simulink model "SecRwRtStArmScrnIsPosChk"  (R2018b)
settings: Solver=FixedStepDiscrete  StartTime=0.0  StopTime=10.0  FixedStep=0.01  RelTol=1e-3
undefined symbols (not defined in the file or in its folder): KeSMSuSecRwStArmTochPosDelta_Val, KeSMSuSecRwStArmTochPosTolr_Val
libraries: simulink x5, StIsPosChkLib x4
settings Model: Creator=sn2xws  LastModifiedBy=sn2xws
settings DataIOCC: SaveFormat=StructureWithTime
settings OptimizationCC: DefaultParameterBehavior=Inlined  EnhancedBackFolding=on  PassReuseOutputArgsAs=Individual arguments  ZeroExternalMemoryAtStartup=off  ZeroInternalMemoryAtStartup=off  OptimizeBlockOrder=speed  DifferentSizesBufferReuse=on  OptimizationCustomize=off
settings DebuggingCC: ParameterTunabilityLossMsg=error
settings ModelReferenceCC: ModelReferenceNumInstancesAllowed=Single
settings SFSimCC: MATLABDynamicMemAlloc=off
settings RTWCC: SystemTargetFile=autosar.tlc  GenCodeOnly=on  TemplateMakefile=ert_default_tmf  Description=AUTOSAR  GenerateReport=on  IncludeHyperlinkInReport=on  LaunchReport=on  GenerateTraceInfo=on  GenerateTraceReport=on  GenerateTraceReportSl=on  GenerateTraceReportSf=on  GenerateTraceReportEml=on
settings CodeAppCC: ForceParamTrailComments=on  IgnoreCustomStorageClasses=off  OperatorAnnotations=on  SimulinkDataObjDesc=on  SFDataObjDesc=on  InsertBlockDesc=on
settings STFCustomTargetCC: TargetLangStandard=C99 (ISO)  MultiwordLength=256  ParMdlRefBuildCompliant=on  CompOptLevelCompliant=on  IncludeMdlTerminateFcn=off  CombineOutputUpdateFcns=on  SuppressErrorStatus=on  ERTCustomFileBanners=on  SupportNonFinite=off  SupportComplex=off  SupportContinuousTime=off  SupportNonInlinedSFcns=off  RemoveResetFunc=on  MATLABClassNameForMDSCustomization=Simulink.SoftwareTarget.ERTCustomization  AutosarCompliant=on  UseToolchainInfoCompliant=on  LookupTableObjectStructAxisOrder=2,1,3,4,...  LUTObjectStructOrderEvenSpacing=Size,Table,Breakpoints  SystemTargetFile=autosar.tlc
settings ERTTargetCC: TargetLangStandard=C99 (ISO)  ConcurrentExecutionCompliant=off  IncludeMdlTerminateFcn=off  SuppressErrorStatus=on  SupportNonFinite=off  SupportComplex=off  ModelStepFunctionPrototypeControlCompliant=off  CPPClassGenCompliant=off  AutosarCompliant=on  LookupTableObjectStructAxisOrder=2,1,3,4,...  LUTObjectStructOrderEvenSpacing=Size,Table,Breakpoints  InlinedParameterPlacement=NonHierarchical  ERTCustomFileTemplate=example_file_process.tlc  ERTFilePackagingFormat=Compact

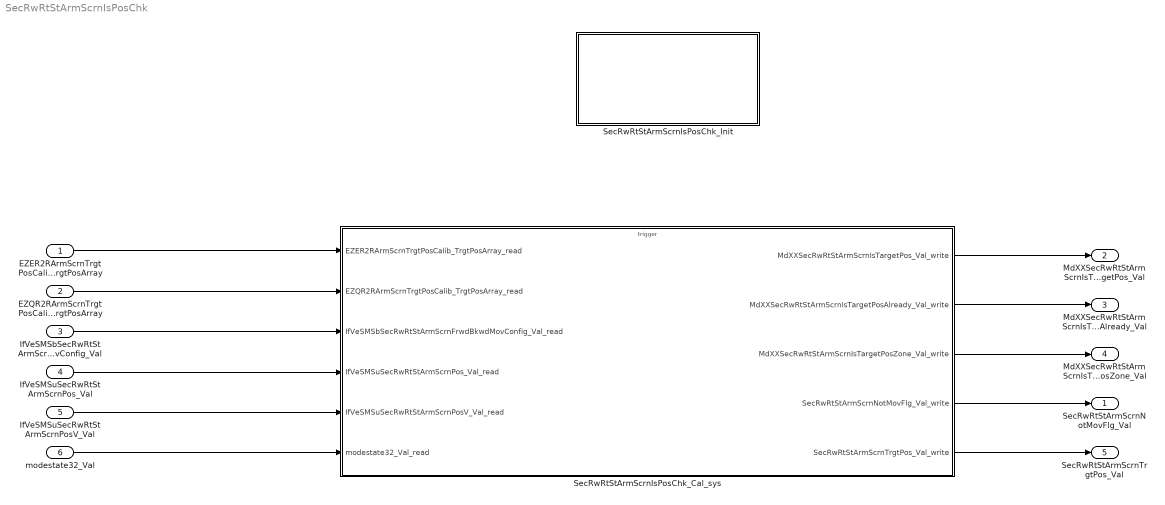
== system SecRwRtStArmScrnIsPosChk ==
  EZER2RArmScrnTrgtPosCalib_TrgtPosArray : Inport  Description=|  OutDataTypeStr=uint16  PortDimensions=3
      | 0:Pos
      | 1:Max
      | 2:Min
  EZQR2RArmScrnTrgtPosCalib_TrgtPosArray : Inport  Description=|  Port=2  OutDataTypeStr=uint16  PortDimensions=3
      | 0:Pos
      | 1:Max
      | 2:Min
  IfVeSMSbSecRwRtStArmScrnFrwdBkwdMovConfig_Val : Inport  Port=3  OutDataTypeStr=boolean  PortDimensions=1
  IfVeSMSuSecRwRtStArmScrnPos_Val : Inport  Port=4  OutDataTypeStr=uint16  PortDimensions=1
  IfVeSMSuSecRwRtStArmScrnPosV_Val : Inport  Port=5  OutDataTypeStr=boolean  PortDimensions=1
  modestate32_Val : Inport  Port=6  OutDataTypeStr=uint32  PortDimensions=1
  SecRwRtStArmScrnIsPosChk_Cal_sys : Subsystem
  SecRwRtStArmScrnIsPosChk_Init : Subsystem
  SecRwRtStArmScrnNotMovFlg_Val : Outport  OutDataTypeStr=boolean  PortDimensions=1
  MdXXSecRwRtStArmScrnIsTargetPos_Val : Outport  Port=2  OutDataTypeStr=uint32  PortDimensions=1
  MdXXSecRwRtStArmScrnIsTargetPosAlready_Val : Outport  Port=3  OutDataTypeStr=uint32  PortDimensions=1
  MdXXSecRwRtStArmScrnIsTargetPosZone_Val : Outport  Port=4  OutDataTypeStr=uint32  PortDimensions=1
  SecRwRtStArmScrnTrgtPos_Val : Outport  Port=5  OutDataTypeStr=uint16  PortDimensions=1
  wires:
  EZER2RArmScrnTrgtPosCalib_TrgtPosArray/1 -> SecRwRtStArmScrnIsPosChk_Cal_sys/1(EZER2RArmScrnTrgtPosCalib_TrgtPosArray_read)
  EZQR2RArmScrnTrgtPosCalib_TrgtPosArray/1 -> SecRwRtStArmScrnIsPosChk_Cal_sys/2(EZQR2RArmScrnTrgtPosCalib_TrgtPosArray_read)
  IfVeSMSbSecRwRtStArmScrnFrwdBkwdMovConfig_Val/1 -> SecRwRtStArmScrnIsPosChk_Cal_sys/3(IfVeSMSbSecRwRtStArmScrnFrwdBkwdMovConfig_Val_read)
  IfVeSMSuSecRwRtStArmScrnPos_Val/1 -> SecRwRtStArmScrnIsPosChk_Cal_sys/4(IfVeSMSuSecRwRtStArmScrnPos_Val_read)
  IfVeSMSuSecRwRtStArmScrnPosV_Val/1 -> SecRwRtStArmScrnIsPosChk_Cal_sys/5(IfVeSMSuSecRwRtStArmScrnPosV_Val_read)
  modestate32_Val/1 -> SecRwRtStArmScrnIsPosChk_Cal_sys/6(modestate32_Val_read)
  SecRwRtStArmScrnIsPosChk_Cal_sys/1(MdXXSecRwRtStArmScrnIsTargetPos_Val_write) -> MdXXSecRwRtStArmScrnIsTargetPos_Val/1
  SecRwRtStArmScrnIsPosChk_Cal_sys/2(MdXXSecRwRtStArmScrnIsTargetPosAlready_Val_write) -> MdXXSecRwRtStArmScrnIsTargetPosAlready_Val/1
  SecRwRtStArmScrnIsPosChk_Cal_sys/3(MdXXSecRwRtStArmScrnIsTargetPosZone_Val_write) -> MdXXSecRwRtStArmScrnIsTargetPosZone_Val/1
  SecRwRtStArmScrnIsPosChk_Cal_sys/4(SecRwRtStArmScrnNotMovFlg_Val_write) -> SecRwRtStArmScrnNotMovFlg_Val/1
  SecRwRtStArmScrnIsPosChk_Cal_sys/5(SecRwRtStArmScrnTrgtPos_Val_write) -> SecRwRtStArmScrnTrgtPos_Val/1

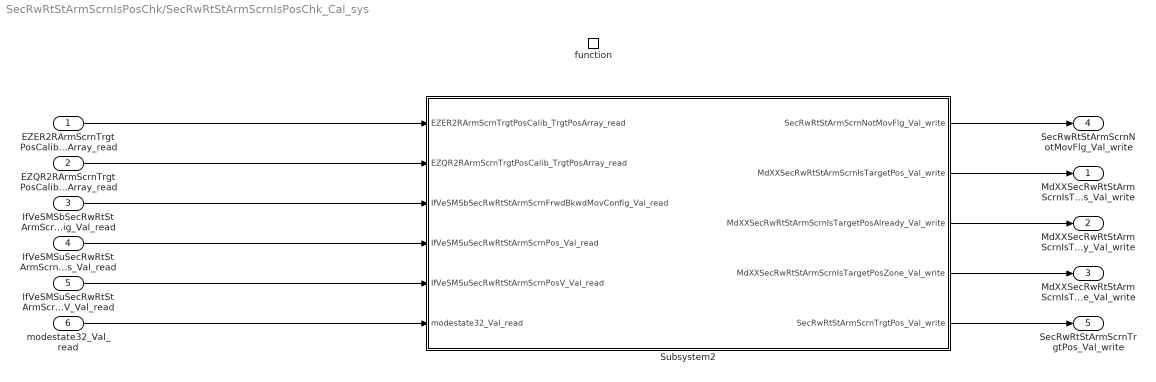
== system SecRwRtStArmScrnIsPosChk/SecRwRtStArmScrnIsPosChk_Cal_sys ==
  EZER2RArmScrnTrgtPosCalib_TrgtPosArray_read : Inport
  EZQR2RArmScrnTrgtPosCalib_TrgtPosArray_read : Inport  Port=2
  IfVeSMSbSecRwRtStArmScrnFrwdBkwdMovConfig_Val_read : Inport  Port=3
  IfVeSMSuSecRwRtStArmScrnPos_Val_read : Inport  Port=4
  IfVeSMSuSecRwRtStArmScrnPosV_Val_read : Inport  Port=5
  modestate32_Val_read : Inport  Port=6
  function : TriggerPort  TriggerType=function-call  IsSimulinkFunction=on  FunctionName=SecRwRtStArmScrnIsPosChk_Cal  VariantControl=(inherit)
  Subsystem2 : Subsystem
  MdXXSecRwRtStArmScrnIsTargetPos_Val_write : Outport
      settings: EnsureOutportIsVirtual=on
  MdXXSecRwRtStArmScrnIsTargetPosAlready_Val_write : Outport  Port=2
      settings: EnsureOutportIsVirtual=on
  MdXXSecRwRtStArmScrnIsTargetPosZone_Val_write : Outport  Port=3
      settings: EnsureOutportIsVirtual=on
  SecRwRtStArmScrnNotMovFlg_Val_write : Outport  Port=4
      settings: EnsureOutportIsVirtual=on
  SecRwRtStArmScrnTrgtPos_Val_write : Outport  Port=5
      settings: EnsureOutportIsVirtual=on
  wires:
  EZER2RArmScrnTrgtPosCalib_TrgtPosArray_read/1 -> Subsystem2/1(EZER2RArmScrnTrgtPosCalib_TrgtPosArray_read)
  EZQR2RArmScrnTrgtPosCalib_TrgtPosArray_read/1 -> Subsystem2/2(EZQR2RArmScrnTrgtPosCalib_TrgtPosArray_read)
  IfVeSMSbSecRwRtStArmScrnFrwdBkwdMovConfig_Val_read/1 -> Subsystem2/3(IfVeSMSbSecRwRtStArmScrnFrwdBkwdMovConfig_Val_read)
  IfVeSMSuSecRwRtStArmScrnPos_Val_read/1 -> Subsystem2/4(IfVeSMSuSecRwRtStArmScrnPos_Val_read)
  IfVeSMSuSecRwRtStArmScrnPosV_Val_read/1 -> Subsystem2/5(IfVeSMSuSecRwRtStArmScrnPosV_Val_read)
  modestate32_Val_read/1 -> Subsystem2/6(modestate32_Val_read)
  Subsystem2/1(SecRwRtStArmScrnNotMovFlg_Val_write) -> SecRwRtStArmScrnNotMovFlg_Val_write/1
  Subsystem2/2(MdXXSecRwRtStArmScrnIsTargetPos_Val_write) -> MdXXSecRwRtStArmScrnIsTargetPos_Val_write/1
  Subsystem2/3(MdXXSecRwRtStArmScrnIsTargetPosAlready_Val_write) -> MdXXSecRwRtStArmScrnIsTargetPosAlready_Val_write/1
  Subsystem2/4(MdXXSecRwRtStArmScrnIsTargetPosZone_Val_write) -> MdXXSecRwRtStArmScrnIsTargetPosZone_Val_write/1
  Subsystem2/5(SecRwRtStArmScrnTrgtPos_Val_write) -> SecRwRtStArmScrnTrgtPos_Val_write/1

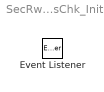
== system SecRwRtStArmScrnIsPosChk/SecRwRtStArmScrnIsPosChk_Init ==
  Event Listener : EventListener  EventName=reset

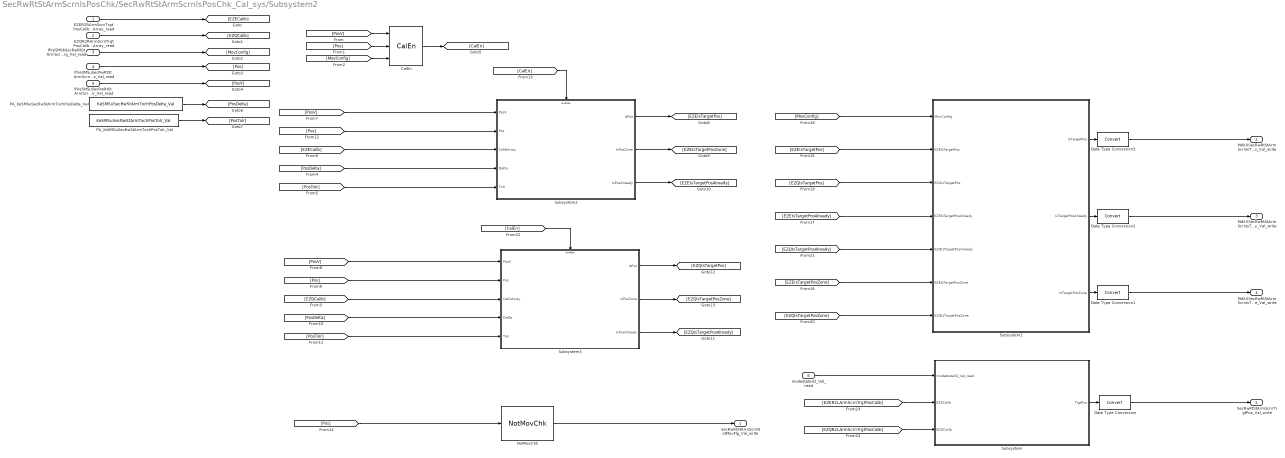
== system SecRwRtStArmScrnIsPosChk/SecRwRtStArmScrnIsPosChk_Cal_sys/Subsystem2 ==
  EZER2RArmScrnTrgtPosCalib_TrgtPosArray_read : Inport
  EZQR2RArmScrnTrgtPosCalib_TrgtPosArray_read : Inport  Port=2
  IfVeSMSbSecRwRtStArmScrnFrwdBkwdMovConfig_Val_read : Inport  Port=3
  IfVeSMSuSecRwRtStArmScrnPos_Val_read : Inport  Port=4
  IfVeSMSuSecRwRtStArmScrnPosV_Val_read : Inport  Port=5
  modestate32_Val_read : Inport  Port=6
  CalEn : StIsPosChkLib/CalEn  SystemSampleTime=-1
  Data Type Conversion{,1..3} (4 alike) : DataTypeConversion
  NotMovChk : StIsPosChkLib/NotMovChk  SystemSampleTime=-1
  PA_KeSMSuSecRwStArmTochPosDelta_Val : Constant  Value=KeSMSuSecRwStArmTochPosDelta_Val
  PA_KeSMSuSecRwStArmTochPosTolr_Val : Constant  Value=KeSMSuSecRwStArmTochPosTolr_Val
  Subsystem : Subsystem
  Subsystem1 : Subsystem
  Subsystem2 : Subsystem
  Subsystem3 : Subsystem
  SecRwRtStArmScrnNotMovFlg_Val_write : Outport
      settings: EnsureOutportIsVirtual=on
  MdXXSecRwRtStArmScrnIsTargetPos_Val_write : Outport  Port=2
      settings: EnsureOutportIsVirtual=on
  MdXXSecRwRtStArmScrnIsTargetPosAlready_Val_write : Outport  Port=3
      settings: EnsureOutportIsVirtual=on
  MdXXSecRwRtStArmScrnIsTargetPosZone_Val_write : Outport  Port=4
      settings: EnsureOutportIsVirtual=on
  SecRwRtStArmScrnTrgtPos_Val_write : Outport  Port=5
      settings: EnsureOutportIsVirtual=on
  wires:
  EZQR2RArmScrnTrgtPosCalib_TrgtPosArray_read/1 -> [EZQCalib]
  [EZQR2LArmScrnTrgtPosCalib] -> Subsystem/3(EZQCalib)
  modestate32_Val_read/1 -> Subsystem/1(modestate32_Val_read)
  [PosDelta] -> Subsystem3/4(Delta)
  [PosV] -> Subsystem2/1(PosV)
  CalEn/1 -> [CalEn]
  [MovConfig] -> CalEn/3
  Subsystem2/3(IsPosAlready) -> [EZEIsTargetPosAlready]
  [PosTolr] -> Subsystem2/5(Tolr)
  Data Type Conversion2/1 -> MdXXSecRwRtStArmScrnIsTargetPosAlready_Val_write/1
  [PosV] -> CalEn/1
  IfVeSMSuSecRwRtStArmScrnPosV_Val_read/1 -> [PosV]
  PA_KeSMSuSecRwStArmTochPosDelta_Val/1 -> [PosDelta]
  [EZQIsTargetPosAlready] -> Subsystem1/5(EZQIsTargetPosAlready)
  IfVeSMSbSecRwRtStArmScrnFrwdBkwdMovConfig_Val_read/1 -> [MovConfig]
  [EZEIsTargetPosZone] -> Subsystem1/6(EZEIsTargetPosZone)
  EZER2RArmScrnTrgtPosCalib_TrgtPosArray_read/1 -> [EZECalib]
  PA_KeSMSuSecRwStArmTochPosTolr_Val/1 -> [PosTolr]
  IfVeSMSuSecRwRtStArmScrnPos_Val_read/1 -> [Pos]
  [PosV] -> Subsystem3/1(PosV)
  Subsystem/1(TrgtPos) -> Data Type Conversion/1
  Subsystem1/2(IsTargetPosAlready) -> Data Type Conversion2/1
  [Pos] -> Subsystem3/2(Pos)
  Subsystem1/1(IsTargetPos) -> Data Type Conversion3/1
  [PosDelta] -> Subsystem2/4(Delta)
  [CalEn] -> Subsystem3/Enable
  Subsystem3/1(IsPos) -> [EZQIsTargetPos]
  [EZQCalib] -> Subsystem3/3(CalibArray)
  Subsystem3/3(IsPosAlready) -> [EZQIsTargetPosAlready]
  Subsystem3/2(IsPosZone) -> [EZQIsTargetPosZone]
  [PosTolr] -> Subsystem3/5(Tolr)
  [EZQIsTargetPos] -> Subsystem1/3(EZQIsTargetPos)
  Subsystem1/3(IsTargetPosZone) -> Data Type Conversion1/1
  Subsystem2/1(IsPos) -> [EZEIsTargetPos]
  [EZEIsTargetPosAlready] -> Subsystem1/4(EZEIsTargetPosAlready)
  Subsystem2/2(IsPosZone) -> [EZEIsTargetPosZone]
  [Pos] -> NotMovChk/1
  [Pos] -> Subsystem2/2(Pos)
  NotMovChk/1 -> SecRwRtStArmScrnNotMovFlg_Val_write/1
  [Pos] -> CalEn/2
  [EZEIsTargetPos] -> Subsystem1/2(EZEIsTargetPos)
  [MovConfig] -> Subsystem1/1(MovConfig)
  [CalEn] -> Subsystem2/Enable
  [EZECalib] -> Subsystem2/3(CalibArray)
  [EZQIsTargetPosZone] -> Subsystem1/7(EZQIsTargetPosZone)
  Data Type Conversion1/1 -> MdXXSecRwRtStArmScrnIsTargetPosZone_Val_write/1
  Data Type Conversion3/1 -> MdXXSecRwRtStArmScrnIsTargetPos_Val_write/1
  [EZER2LArmScrnTrgtPosCalib] -> Subsystem/2(EZECalib)
  Data Type Conversion/1 -> SecRwRtStArmScrnTrgtPos_Val_write/1

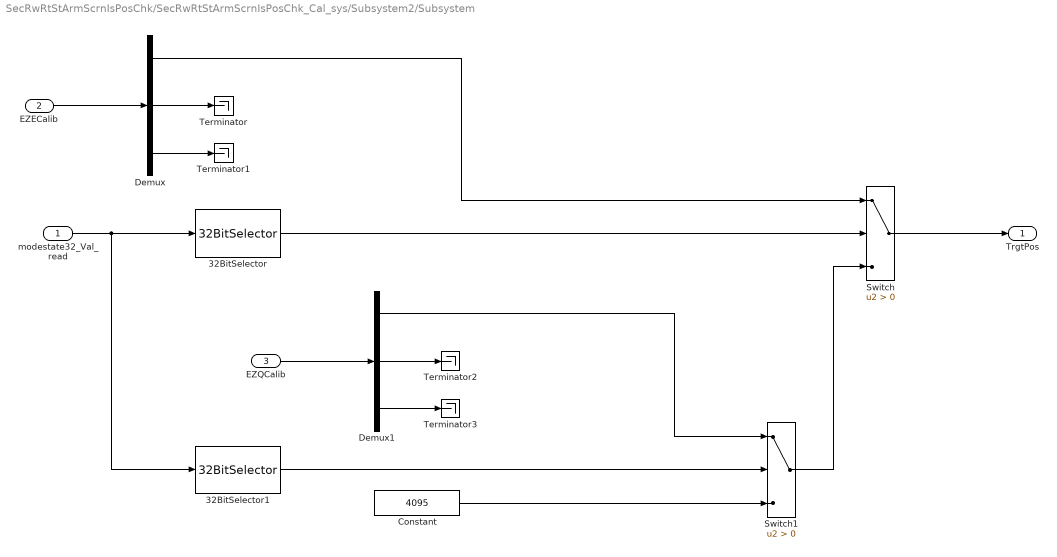
== system SecRwRtStArmScrnIsPosChk/SecRwRtStArmScrnIsPosChk_Cal_sys/Subsystem2/Subsystem ==
  modestate32_Val_read : Inport
  EZECalib : Inport  Port=2
  EZQCalib : Inport  Port=3
  32BitSelector : StIsPosChkLib/32BitSelector  BitNum=0
  32BitSelector1 : StIsPosChkLib/32BitSelector  BitNum=3
  Constant : Constant  Value=4095  OutDataTypeStr=uint16
  Demux : Demux  Outputs=3
  Demux1 : Demux  Outputs=3
  Switch : Switch  Criteria=u2 > Threshold
  Switch1 : Switch  Criteria=u2 > Threshold
  Terminator{,1..3} (4 alike) : Terminator
  TrgtPos : Outport
      settings: EnsureOutportIsVirtual=on
  wires:
  32BitSelector/1 -> Switch/2
  modestate32_Val_read/1 -> 32BitSelector1/1, 32BitSelector/1
  Demux/1 -> Switch/1
  Demux/3 -> Terminator1/1
  Demux/2 -> Terminator/1
  EZECalib/1 -> Demux/1
  EZQCalib/1 -> Demux1/1
  Demux1/2 -> Terminator2/1
  Demux1/3 -> Terminator3/1
  Demux1/1 -> Switch1/1
  Switch/1 -> TrgtPos/1
  Switch1/1 -> Switch/3
  32BitSelector1/1 -> Switch1/2
  Constant/1 -> Switch1/3

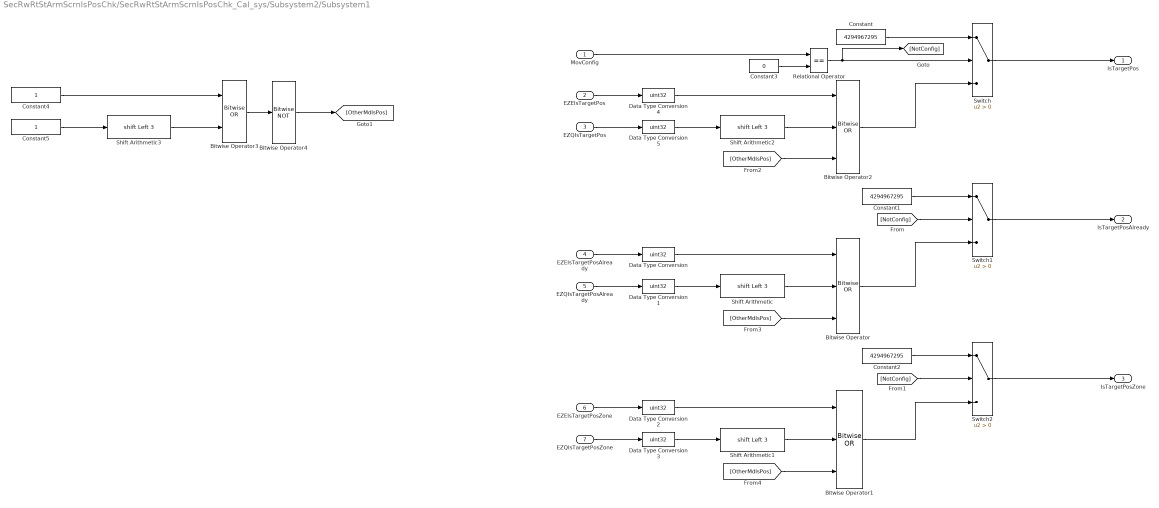
== system SecRwRtStArmScrnIsPosChk/SecRwRtStArmScrnIsPosChk_Cal_sys/Subsystem2/Subsystem1 ==
  MovConfig : Inport
  EZEIsTargetPos : Inport  Port=2
  EZQIsTargetPos : Inport  Port=3
  EZEIsTargetPosAlready : Inport  Port=4
  EZQIsTargetPosAlready : Inport  Port=5
  EZEIsTargetPosZone : Inport  Port=6
  EZQIsTargetPosZone : Inport  Port=7
  Bitwise Operator : simulink/Logic and Bit Operations/Bitwise Operator  logicop=OR  UseBitMask=off  NumInputPorts=3  BitMask=bin2dec('11011001')  BitMaskRealWorld=Stored Integer
  Bitwise Operator1 : simulink/Logic and Bit Operations/Bitwise Operator  logicop=OR  UseBitMask=off  NumInputPorts=3  BitMask=bin2dec('11011001')  BitMaskRealWorld=Stored Integer
  Bitwise Operator2 : simulink/Logic and Bit Operations/Bitwise Operator  logicop=OR  UseBitMask=off  NumInputPorts=3  BitMask=bin2dec('11011001')  BitMaskRealWorld=Stored Integer
  Bitwise Operator3 : simulink/Logic and Bit Operations/Bitwise Operator  logicop=OR  UseBitMask=off  NumInputPorts=2  BitMask=bin2dec('11011001')  BitMaskRealWorld=Stored Integer
  Bitwise Operator4 : simulink/Logic and Bit Operations/Bitwise Operator  logicop=NOT  UseBitMask=off  BitMask=bin2dec('11011001')  BitMaskRealWorld=Stored Integer
  Constant : Constant  Value=4294967295  OutDataTypeStr=uint32
  Constant1 : Constant  Value=4294967295  OutDataTypeStr=uint32
  Constant2 : Constant  Value=4294967295  OutDataTypeStr=uint32
  Constant3 : Constant  Value=0  OutDataTypeStr=uint8
  Constant4 : Constant  OutDataTypeStr=uint32
  Constant5 : Constant  OutDataTypeStr=uint32
  Data Type Conversion{,1..5} (6 alike) : DataTypeConversion  OutDataTypeStr=uint32
  Relational Operator : RelationalOperator  Operator===  OutDataTypeStr=boolean  RndMeth=Simplest
  Shift Arithmetic{,1..3} (4 alike) : ArithShift  BitShiftNumber=3  BitShiftDirection=Left
  Switch : Switch  Criteria=u2 > Threshold
  Switch1 : Switch  Criteria=u2 > Threshold
  Switch2 : Switch  Criteria=u2 > Threshold
  IsTargetPos : Outport
      settings: EnsureOutportIsVirtual=on
  IsTargetPosAlready : Outport  Port=2
      settings: EnsureOutportIsVirtual=on
  IsTargetPosZone : Outport  Port=3
      settings: EnsureOutportIsVirtual=on
  wires:
  Constant3/1 -> Relational Operator/2
  Constant/1 -> Switch/1
  Relational Operator/1 -> [NotConfig], Switch/2
  MovConfig/1 -> Relational Operator/1
  Switch/1 -> IsTargetPos/1
  [NotConfig] -> Switch1/2
  Constant1/1 -> Switch1/1
  Switch1/1 -> IsTargetPosAlready/1
  Switch2/1 -> IsTargetPosZone/1
  Constant2/1 -> Switch2/1
  [NotConfig] -> Switch2/2
  Data Type Conversion1/1 -> Shift Arithmetic/1
  Data Type Conversion/1 -> Bitwise Operator/1
  Shift Arithmetic/1 -> Bitwise Operator/2
  Shift Arithmetic1/1 -> Bitwise Operator1/2
  Data Type Conversion2/1 -> Bitwise Operator1/1
  Data Type Conversion3/1 -> Shift Arithmetic1/1
  Bitwise Operator1/1 -> Switch2/3
  Bitwise Operator/1 -> Switch1/3
  Shift Arithmetic2/1 -> Bitwise Operator2/2
  Data Type Conversion4/1 -> Bitwise Operator2/1
  Data Type Conversion5/1 -> Shift Arithmetic2/1
  Bitwise Operator2/1 -> Switch/3
  EZEIsTargetPos/1 -> Data Type Conversion4/1
  EZQIsTargetPos/1 -> Data Type Conversion5/1
  EZQIsTargetPosZone/1 -> Data Type Conversion3/1
  EZEIsTargetPosZone/1 -> Data Type Conversion2/1
  EZQIsTargetPosAlready/1 -> Data Type Conversion1/1
  EZEIsTargetPosAlready/1 -> Data Type Conversion/1
  Constant4/1 -> Bitwise Operator3/1
  Shift Arithmetic3/1 -> Bitwise Operator3/2
  Constant5/1 -> Shift Arithmetic3/1
  Bitwise Operator3/1 -> Bitwise Operator4/1
  Bitwise Operator4/1 -> [OtherMdIsPos]
  [OtherMdIsPos] -> Bitwise Operator2/3
  [OtherMdIsPos] -> Bitwise Operator/3
  [OtherMdIsPos] -> Bitwise Operator1/3

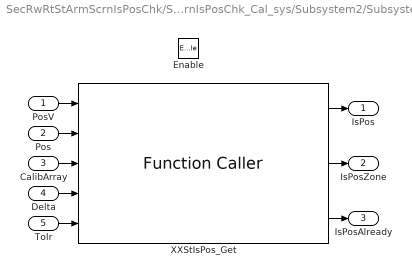
== system SecRwRtStArmScrnIsPosChk/SecRwRtStArmScrnIsPosChk_Cal_sys/Subsystem2/Subsystem2 ==
  PosV : Inport
  Pos : Inport  Port=2
  CalibArray : Inport  Port=3
  Delta : Inport  Port=4
  Tolr : Inport  Port=5
  Enable : EnablePort
  XXStIsPos_Get : FunctionCaller  FunctionPrototype=[IsPos,IsPosZone,IsPosAlready] = XXStIsPos_Get(PosV,Pos,CalibArray,Delta,Tolr)  InputArgumentSpecifications=boolean(true), uint16(1), uint16([1;1;1]), uint16(1), uint16(1)  OutputArgumentSpecifications=boolean(true), boolean(true), boolean(true)
  IsPos : Outport
  IsPosZone : Outport  Port=2
  IsPosAlready : Outport  Port=3
  wires:
  CalibArray/1 -> XXStIsPos_Get/3
  PosV/1 -> XXStIsPos_Get/1
  XXStIsPos_Get/1 -> IsPos/1
  Pos/1 -> XXStIsPos_Get/2
  XXStIsPos_Get/3 -> IsPosAlready/1
  XXStIsPos_Get/2 -> IsPosZone/1
  Delta/1 -> XXStIsPos_Get/4
  Tolr/1 -> XXStIsPos_Get/5

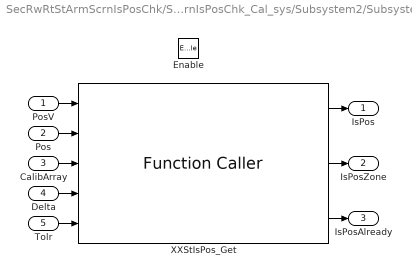
== system SecRwRtStArmScrnIsPosChk/SecRwRtStArmScrnIsPosChk_Cal_sys/Subsystem2/Subsystem3 ==
  PosV : Inport
  Pos : Inport  Port=2
  CalibArray : Inport  Port=3
  Delta : Inport  Port=4
  Tolr : Inport  Port=5
  Enable : EnablePort
  XXStIsPos_Get : FunctionCaller  FunctionPrototype=[IsPos,IsPosZone,IsPosAlready] = XXStIsPos_Get(PosV,Pos,CalibArray,Delta,Tolr)  InputArgumentSpecifications=boolean(true), uint16(1), uint16([1;1;1]), uint16(1), uint16(1)  OutputArgumentSpecifications=boolean(true), boolean(true), boolean(true)
  IsPos : Outport
  IsPosZone : Outport  Port=2
  IsPosAlready : Outport  Port=3
  wires:
  CalibArray/1 -> XXStIsPos_Get/3
  PosV/1 -> XXStIsPos_Get/1
  XXStIsPos_Get/1 -> IsPos/1
  Pos/1 -> XXStIsPos_Get/2
  XXStIsPos_Get/3 -> IsPosAlready/1
  XXStIsPos_Get/2 -> IsPosZone/1
  Delta/1 -> XXStIsPos_Get/4
  Tolr/1 -> XXStIsPos_Get/5
